simulink model "commhdlQPSKTxRxLoopback"  (R2025b)
settings: Solver=FixedStepDiscrete  StartTime=0.0  StopTime=stopTime  RelTol=1e-3
PostLoadFcn:
  | hScopeConfig = get_param([gcs '/Receiver/QPSK Rx/Frequency and Time Synchronizer/Symbol Synchronizer/No HDL/QPSK Receiver Eye Diagram'],'ScopeConfiguration');
  | 
  | hScopeConfig.OpenAtSimulationStart = false;
  | hScopeConfig.Visible = false;
  | SamplesPerSymbol = 4;
  | %UpsamplesRx = 1;
  | clear hScopeConfig
InitFcn:
  | commhdlQPSKTxRxModelInit;
  | % Rate bridge: ADRV9002/Jupiter radio runs at 15.36 MHz = 2x the 7.68 MHz
  | % (4 samples/symbol @ Rsym=1.92 MHz) the QPSK Rx requires. The deployed
  | % Receiver must downsample the ADC stream by 2. UpsamplesRx=1 fed the QPSK
  | % Rx 8 sps (2x-upsampled) and broke symbol sync / the loopback bit check.
  | UpsamplesRx = 2;
  | UpsamplesTx = 1;
  | clear simTimingOffset;
StopFcn:
  | if exist('simTimingOffset','var')
  |   disp('Simulation completed');
  |   %QPSKTxRxVerification;
  | end
values from neighbouring files (symbols this model uses):
  Rsym = variant{2}    [BandwidthVariantSimTest.m]    (also in CoarseFreqEstimatorTest.m = CoarseFreqEstimatorTest.Rsym; PreambleDetectorTest.m = 1920000)
undefined symbols (not defined in the file or in its folder): Add, Config, fsym, randsrc, RandStream, Shift
libraries: hdlsllib x149, simulink x40, dspsigops x36, dsphdlfiltering2 x6, dsphdlsigops2 x4, dsphdlmathfun2 x4, commdigbbndpm3 x4, commchan3 x1, commrflib2 x1
(part 6 of 6)

== system commhdlQPSKTxRxLoopback/TxRxLoopback/Receiver/QPSK Rx/Frequency and Time Synchronizer/Coarse Frequency Compensator/Coarse Frequency Estimator/Integrator ==
  note: store the value in the Reg before reset
  dataIn : Inport
  validIn : Inport  Port=2
  Add1 : Sum  Inputs=|++  OutDataTypeStr=Inherit: Same as first input
  Delay : Delay  DelayLength=1
  Delay1 : Delay  DelayLength=1
  Delay2 : Delay  DelayLength=1
  Integ Reg : hdlsllib/Discrete/Unit Delay Enabled Resettable Synchronous  InitialCondition=0.0  SampleTime=-1
  Reset Generator : Subsystem
  Store Reg : hdlsllib/Discrete/Unit Delay Enabled Synchronous  InitialCondition=0.0  SampleTime=-1
  IntegOut : Outport
  IntegValid : Outport  Port=2
  wires:
  Delay2/1 -> Integ Reg/2
  Reset Generator/1(reset) -> Integ Reg/3, Store Reg/2, Delay/1
  Store Reg/1 -> IntegOut/1
  Delay/1 -> IntegValid/1
  Delay1/1 -> Add1/1
  dataIn/1 -> Delay1/1
  validIn/1 -> Reset Generator/1(validIn), Delay2/1
  Integ Reg/1 -> Add1/2, Store Reg/1
  Add1/1 -> Integ Reg/1

== system commhdlQPSKTxRxLoopback/TxRxLoopback/Receiver/QPSK Rx/Frequency and Time Synchronizer/Phase Ambiguity Estimation and Correction/Phase Ambiguity Corrector/Reciprocal ==
  dataIn : Inport
  Compare To Constant : simulink/Logic and Bit Operations/Compare To Constant  relop=<  const=0  OutDataTypeStr=boolean
  Data Type Conversion : DataTypeConversion  OutDataTypeStr=fixdt(1,WL,0)  ConvertRealWorld=Stored Integer (SI)  SaturateOnIntegerOverflow=off  RndMeth=Floor
  Data Type Conversion1 : DataTypeConversion  OutDataTypeStr=fixdt(0,LUTAddrWL,0)  ConvertRealWorld=Stored Integer (SI)  SaturateOnIntegerOverflow=off  RndMeth=Floor
  Data Type Conversion2 : DataTypeConversion  OutDataTypeStr=fixdt(0,WL-LUTAddrWL,0)  ConvertRealWorld=Stored Integer (SI)  SaturateOnIntegerOverflow=off  RndMeth=Floor
  Delay : Delay  DelayLength=1
  Delay1 : Delay  DelayLength=1
  Delay2 : Delay  DelayLength=1
  Extract Bits : simulink/Logic and Bit Operations/Extract Bits  bitsToExtract=Range ending with least significant bit  numBits=LUTAddrWL  bitIdxRange=[0 7]  outScalingMode=Treat bit field as an integer
  Function Impl : Subsystem
  dataOut : Outport
  wires:
  Data Type Conversion2/1 -> Function Impl/1(switch)
  Delay2/1 -> Data Type Conversion1/1
  Delay1/1 -> Data Type Conversion2/1
  Delay/1 -> Extract Bits/1, Compare To Constant/1
  Function Impl/1(functionValues) -> dataOut/1
  Data Type Conversion1/1 -> Function Impl/2(LUTAddr)
  Compare To Constant/1 -> Delay1/1
  Data Type Conversion/1 -> Delay/1
  Extract Bits/1 -> Delay2/1
  dataIn/1 -> Data Type Conversion/1

== system commhdlQPSKTxRxLoopback/TxRxLoopback/Receiver/QPSK Rx/Frequency and Time Synchronizer/Phase Ambiguity Estimation and Correction/Phase Ambiguity Estimator/Subsystem ==
  L : Inport
  H : Inport  Port=2
  Delay6 : Delay  DelayLength=1  InitialCondition=1
  Logical Operator : Logic  AllPortsSameDT=off  OutDataTypeStr=boolean
  Logical Operator1 : Logic  Operator=NOT  IconShape=distinctive  AllPortsSameDT=off  OutDataTypeStr=boolean
  Logical Operator2 : Logic  Operator=OR  AllPortsSameDT=off  OutDataTypeStr=boolean
  Out2 : Outport
  wires:
  Logical Operator2/1 -> Delay6/1
  Logical Operator/1 -> Logical Operator2/2
  Logical Operator1/1 -> Logical Operator/1
  Delay6/1 -> Logical Operator/2, Out2/1
  H/1 -> Logical Operator2/1
  L/1 -> Logical Operator1/1

== system commhdlQPSKTxRxLoopback/TxRxLoopback/Receiver/QPSK Rx/Frequency and Time Synchronizer/Phase Ambiguity Estimation and Correction/Phase Ambiguity Estimator/Subsystem1 ==
  In1 : Inport
  validIn : Inport  Port=2
  Logical Operator1 : Logic  IconShape=distinctive  AllPortsSameDT=off  OutDataTypeStr=boolean
  Logical Operator2 : Logic  Operator=NOT  IconShape=distinctive  AllPortsSameDT=off  OutDataTypeStr=boolean
  validOut : Outport
  wires:
  Logical Operator2/1 -> Logical Operator1/1
  Logical Operator1/1 -> validOut/1
  validIn/1 -> Logical Operator1/2
  In1/1 -> Logical Operator2/1

== system commhdlQPSKTxRxLoopback/TxRxLoopback/Receiver/QPSK Rx/Frequency and Time Synchronizer/Preamble Detector/Correlator/Magnitude Squared ==
  In1 : Inport
  Delay1 : Delay
  Delay2 : Delay
  Delay3 : Delay
  Math Function : Math  Operator=conj
  Product : Product
  Out1 : Outport
  wires:
  Delay3/1 -> Out1/1
  Delay1/1 -> Product/2
  Delay2/1 -> Product/1
  Product/1 -> Delay3/1
  Math Function/1 -> Delay1/1
  In1/1 -> Delay2/1, Math Function/1

== system commhdlQPSKTxRxLoopback/TxRxLoopback/Receiver/QPSK Rx/Frequency and Time Synchronizer/Preamble Detector/Correlator/Magnitude Squared and Moving Sum ==
  scaled1 : Inport
  validIn : Inport  Port=2
  Add : Sum  Inputs=|+-  OutDataTypeStr=Inherit: Same as first input
  Add1 : Sum  Inputs=|++  OutDataTypeStr=Inherit: Same as first input
  Complex to Real-Imag1 : ComplexToRealImag  Output=Real
  Delay : Delay  DelayLength=13  ShowEnablePort=on
      settings: InputPortMap=u0,e6
  Delay{1..4,6,8..10,12} (9 alike) : Delay
  Delay11 : Delay  DelayLength=11
  Delay14 : Delay  DelayLength=1  ShowEnablePort=on
      settings: InputPortMap=u0,e6
  Delay5 : Delay  DelayLength=1
  Delay7 : Delay  DelayLength=1
  Gain : Gain  Gain=ThresoldGainFac  OutDataTypeStr=Inherit: Same as input
  Math Function1 : Math  Operator=conj
  Product1 : Product
  E1 : Outport
  wires:
  Delay12/1 -> Delay10/1
  Delay10/1 -> Delay9/1
  Delay9/1 -> Delay8/1
  Delay8/1 -> Delay7/1, Delay/2
  Delay7/1 -> Delay14/2
  Delay5/1 -> Add1/1
  Delay4/1 -> Add/1, Delay/1
  Delay3/1 -> Gain/1
  Delay2/1 -> Complex to Real-Imag1/1
  Delay1/1 -> Product1/2
  Delay6/1 -> Product1/1
  Gain/1 -> Delay4/1
  Product1/1 -> Delay2/1
  Math Function1/1 -> Delay1/1
  scaled1/1 -> Math Function1/1, Delay6/1
  Delay11/1 -> E1/1
  Add1/1 -> Delay14/1, Delay11/1
  Complex to Real-Imag1/1 -> Delay3/1
  Delay14/1 -> Add1/2
  Delay/1 -> Add/2
  validIn/1 -> Delay12/1
  Add/1 -> Delay5/1

== system commhdlQPSKTxRxLoopback/TxRxLoopback/Receiver/QPSK Rx/Frequency and Time Synchronizer/Preamble Detector/FIFO/Validate Input Push Pop ==
  rst : Inport
  push : Inport  Port=2
  pop : Inport  Port=3
  Compare To Constant : hdlsllib/Logic and Bit Operations/Compare To Constant  relop===  const=0  OutDataTypeStr=boolean
  Compare To Constant1 : hdlsllib/Logic and Bit Operations/Compare To Constant  relop===  const=fifoSize  OutDataTypeStr=boolean
  Constant : Constant  Value=true  SampleTime=-1
  Constant1 : Constant  Value=false  SampleTime=-1
  Delay : Delay  DelayLength=1
  Logical Operator1 : Logic  Operator=XOR  AllPortsSameDT=off  OutDataTypeStr=boolean
  Logical Operator2 : Logic  Operator=NOT  AllPortsSameDT=off  OutDataTypeStr=boolean
  Logical Operator{3..5,7,9} (5 alike) : Logic  AllPortsSameDT=off  OutDataTypeStr=boolean
  Logical Operator6 : Logic  Operator=NOT  AllPortsSameDT=off  OutDataTypeStr=boolean
  Logical Operator8 : Logic  Operator=NOT  AllPortsSameDT=off  OutDataTypeStr=boolean
  MATLAB Function : MATLAB Function  TreatAsAtomicUnit=on  mask{initVal=0, countToVal=fifoSize}
      mask prompts: initVal "Initial value:"; countToVal "Count to value:"
  No HDL : Subsystem
  Switch : Switch  Criteria=u2 ~= 0  SaturateOnIntegerOverflow=off  InputSameDT=off
  valid push : Outport
  valid pop : Outport  Port=2
  numEntries : Outport  Port=3
  wires:
  Delay/1 -> Compare To Constant/1, numEntries/1, Compare To Constant1/1
  rst/1 -> MATLAB Function/1(rst)
  Compare To Constant/1 -> Logical Operator3/1
  pop/1 -> Logical Operator7/1, Logical Operator3/2
  Switch/1 -> MATLAB Function/3(dir)
  MATLAB Function/1(count) -> Delay/1
  Constant1/1 -> Switch/1
  Logical Operator3/1 -> Logical Operator6/1, No HDL/2(popEmptyFIFO)  "pop on empty FIFO"
  Logical Operator4/1 -> Logical Operator2/1, No HDL/1(pushFullFIFO)  "push on full FIFO"
  Constant/1 -> Switch/3
  Compare To Constant1/1 -> Logical Operator4/2
  Logical Operator7/1 -> Logical Operator1/2, Logical Operator8/1, valid pop/1, Switch/2
  Logical Operator6/1 -> Logical Operator7/2
  Logical Operator1/1 -> MATLAB Function/2(enb)
  push/1 -> Logical Operator9/1, Logical Operator5/1
  Logical Operator8/1 -> Logical Operator5/2
  Logical Operator5/1 -> Logical Operator4/1
  Logical Operator2/1 -> Logical Operator9/2
  Logical Operator9/1 -> valid push/1, Logical Operator1/1

== system commhdlQPSKTxRxLoopback/TxRxLoopback/Receiver/QPSK Rx/Frequency and Time Synchronizer/Preamble Detector/Timing Adjust/No HDL ==
  note: This subsystem generates variables required for QPSKRxVerification for validation
  validIn : Inport
  timingOffset : Inport  Port=2
  syncPulse : Inport  Port=3
  Compare To Constant : simulink/Logic and Bit Operations/Compare To Constant  relop===  const=0  OutDataTypeStr=boolean
  Delay : Delay  DelayLength=4
  Delay1 : Delay  DelayLength=4
  Frame Counter : hdlsllib/Sources/HDL Counter  CountType=Free running  CountInit=0  CountStep=1  CountMax=bitsPerPacket/2 - 1  CountFromType=Initial value  CountFrom=0  CountResetPort=off  CountLoadPort=off  CountEnbPort=on  CountDirPort=off  CountHitOutputPort=off  CountDataType=Unsigned  CountWordLen=32  CountFracLen=0  CountSampTime=1
  Logical Operator : Logic  AllPortsSameDT=off  OutDataTypeStr=boolean
  No HDL : Subsystem
  No HDL1 : Subsystem
  Symbol Counter : hdlsllib/Sources/HDL Counter  CountType=Count limited  CountInit=0  CountStep=1  CountMax=bitsPerPacket/2 - 1  CountFromType=Initial value  CountFrom=0  CountResetPort=off  CountLoadPort=off  CountEnbPort=on  CountDirPort=off  CountHitOutputPort=off  CountDataType=Unsigned  CountWordLen=nextpow2(bitsPerPacket/2 - 1)  CountFracLen=0  CountSampTime=1
  Unit Delay Enabled Synchronous : hdlsllib/Discrete/Unit Delay Enabled Synchronous  InitialCondition=0.0  SampleTime=-1
  wires:
  Delay1/1 -> No HDL/1(timingOffset)
  Delay/1 -> No HDL1/Enable, No HDL/Enable
  Unit Delay Enabled Synchronous/1 -> No HDL1/1(frameNumber)
  syncPulse/1 -> Delay/1
  Frame Counter/1 -> Unit Delay Enabled Synchronous/1
  Compare To Constant/1 -> Logical Operator/1
  Logical Operator/1 -> Frame Counter/1, Unit Delay Enabled Synchronous/2
  Symbol Counter/1 -> Compare To Constant/1
  validIn/1 -> Symbol Counter/1, Logical Operator/2
  timingOffset/1 -> Delay1/1

== system commhdlQPSKTxRxLoopback/TxRxLoopback/Receiver/QPSK Rx/Frequency and Time Synchronizer/Symbol Synchronizer/Gardner TED/GTED ==
  In1 : Inport
  Add : Sum
  Add1 : Sum  Inputs=+-
  Add2 : Sum  Inputs=+-
  Complex to Real-Imag : ComplexToRealImag
  Delay{,1..7} (8 alike) : Delay  DelayLength=1
  Delay{8..13} (6 alike) : Delay
  Product : Product
  Product1 : Product
  Out1 : Outport
  wires:
  Delay13/1 -> Add/2
  Delay12/1 -> Product1/2
  Delay11/1 -> Product1/1
  Delay10/1 -> Add/1
  Delay9/1 -> Product/2
  Delay8/1 -> Product/1
  Complex to Real-Imag/2 -> Delay4/1, Add2/2
  Delay7/1 -> Add2/1
  Delay4/1 -> Delay5/1
  Delay6/1 -> Delay7/1
  Add2/1 -> Delay12/1
  Delay5/1 -> Delay6/1, Delay11/1
  Delay1/1 -> Delay8/1, Delay2/1
  Add1/1 -> Delay9/1
  Delay2/1 -> Delay3/1
  Delay/1 -> Delay1/1
  Delay3/1 -> Add1/1
  Complex to Real-Imag/1 -> Delay/1, Add1/2
  In1/1 -> Complex to Real-Imag/1
  Add/1 -> Out1/1
  Product1/1 -> Delay13/1
  Product/1 -> Delay10/1

== system commhdlQPSKTxRxLoopback/TxRxLoopback/Receiver/QPSK Rx/Frequency and Time Synchronizer/Symbol Synchronizer/No HDL/No HDL ==
  data : Inport
  Enable : EnablePort
  Data Type Conversion : DataTypeConversion  OutDataTypeStr=double  SaturateOnIntegerOverflow=off  RndMeth=Floor
  wires:
  data/1 -> Data Type Conversion/1
  Data Type Conversion/1 -> ?

== system commhdlQPSKTxRxLoopback/TxRxLoopback/Receiver/QPSK Rx/Frequency and Time Synchronizer/Symbol Synchronizer/Rate Handle/FIFO ==
  in : Inport
  push : Inport  Port=2
  pop : Inport  Port=3
  reset : Inport  Port=4
  Delay1 : Delay  DelayLength=1
  Pop Counter : hdlsllib/Sources/HDL Counter  CountType=Count limited  CountInit=0  CountStep=1  CountMax=fifoSize -1  CountFromType=Initial value  CountFrom=0  CountResetPort=on  CountLoadPort=off  CountEnbPort=on  CountDirPort=off  CountHitOutputPort=off  CountDataType=Unsigned  CountWordLen=nextpow2(fifoSize)  CountFracLen=0  CountSampTime=1
  Push Counter : hdlsllib/Sources/HDL Counter  CountType=Count limited  CountInit=0  CountStep=1  CountMax=fifoSize -1  CountFromType=Initial value  CountFrom=0  CountResetPort=on  CountLoadPort=off  CountEnbPort=on  CountDirPort=off  CountHitOutputPort=off  CountDataType=Unsigned  CountWordLen=nextpow2(fifoSize)  CountFracLen=0  CountSampTime=1
  Simple Dual Port RAM : hdlsllib/HDL RAMs/Simple Dual Port RAM  ram_size=nextpow2(fifoSize)
  Validate Input Push Pop : Subsystem
  out : Outport
  numEntries : Outport  Port=2
  validPop : Outport  Port=3
  wires:
  Validate Input Push Pop/3(numEntries) -> numEntries/1
  Simple Dual Port RAM/1 -> out/1
  Push Counter/1 -> Simple Dual Port RAM/2
  Pop Counter/1 -> Simple Dual Port RAM/4
  push/1 -> Validate Input Push Pop/2(push)
  pop/1 -> Validate Input Push Pop/3(pop)
  Validate Input Push Pop/1(valid push) -> Simple Dual Port RAM/3, Push Counter/2
  Validate Input Push Pop/2(valid pop) -> validPop/1, Pop Counter/2
  reset/1 -> Delay1/1, Validate Input Push Pop/1(rst)
  in/1 -> Simple Dual Port RAM/1
  Delay1/1 -> Pop Counter/1, Push Counter/1

== system commhdlQPSKTxRxLoopback/TxRxLoopback/Transmitter/QPSK Tx/Bit Packetizer/Data Bits FIFO/No HDL/No HDL ==
  push : Inport
  full : Inport  Port=2
  ncount : Inport  Port=3
  empty : Inport  Port=4
  pop : Inport  Port=5
  Assertion : Assertion
  Assertion1 : Assertion
  Display : Display
  Logical Operator : Logic  Operator=NAND  AllPortsSameDT=off  OutDataTypeStr=boolean
  Logical Operator1 : Logic  Operator=NAND  AllPortsSameDT=off  OutDataTypeStr=boolean
  wires:
  push/1 -> Logical Operator/1
  empty/1 -> Logical Operator1/1
  full/1 -> Logical Operator/2
  pop/1 -> Logical Operator1/2
  Logical Operator/1 -> Assertion/1
  ncount/1 -> Display/1
  Logical Operator1/1 -> Assertion1/1

== system commhdlQPSKTxRxLoopback/Receiver/QPSK Rx/Frequency and Time Synchronizer/Symbol Synchronizer/Rate Handle/FIFO/Validate Input Push Pop/No HDL ==
  pushFullFIFO : Inport
  popEmptyFIFO : Inport  Port=2
  Constant2 : Constant  Value=pushFullDiag  SampleTime=-1
  Constant3 : Constant  Value=popEmptyDiag  SampleTime=-1
  MATLAB Function : MATLAB Function  TreatAsAtomicUnit=on
  wires:
  Constant2/1 -> MATLAB Function/1(pushFullDiag)
  Constant3/1 -> MATLAB Function/2(popEmptyDiag)
  popEmptyFIFO/1 -> MATLAB Function/4(popEmpty)
  pushFullFIFO/1 -> MATLAB Function/3(pushFull)

== system commhdlQPSKTxRxLoopback/TxRxLoopback/Receiver/QPSK Rx/Frequency and Time Synchronizer/Coarse Frequency Compensator/Coarse Frequency Estimator/Integrator/Reset Generator ==
  validIn : Inport
  Compare To Constant : simulink/Logic and Bit Operations/Compare To Constant  relop===  const=integAvgLen  OutDataTypeStr=boolean
  Delay1 : Delay  DelayLength=1
  Delay5 : Delay  DelayLength=1
  HDL Counter : hdlsllib/Sources/HDL Counter  CountType=Count limited  CountInit=0  CountStep=1  CountMax=integAvgLen  CountFromType=Initial value  CountFrom=0  CountResetPort=off  CountLoadPort=off  CountEnbPort=on  CountDirPort=off  CountHitOutputPort=off  CountDataType=Unsigned  CountWordLen=nextpow2(integAvgLen + 1)  CountFracLen=0  CountSampTime=1
  Logical Operator : Logic  AllPortsSameDT=off  OutDataTypeStr=boolean
  reset : Outport
  wires:
  HDL Counter/1 -> Delay5/1
  Compare To Constant/1 -> Logical Operator/2
  validIn/1 -> Delay1/1, HDL Counter/1
  Logical Operator/1 -> reset/1
  Delay5/1 -> Compare To Constant/1
  Delay1/1 -> Logical Operator/1

== system commhdlQPSKTxRxLoopback/TxRxLoopback/Receiver/QPSK Rx/Frequency and Time Synchronizer/Phase Ambiguity Estimation and Correction/Phase Ambiguity Corrector/Reciprocal/Function Impl ==
  switch : Inport
  LUTAddr : Inport  Port=2
  Delay{6..8,10,15..16} (6 alike) : Delay
  Delay9 : Delay  DelayLength=1
  LUT1 : LookupNDDirect  NumberOfTableDimensions=1  Table=LUT(:,1)  DiagnosticForOutOfRangeInput=Error
  LUT2 : LookupNDDirect  NumberOfTableDimensions=1  Table=LUT(:,2)  DiagnosticForOutOfRangeInput=Error
  Multiport Switch : MultiPortSwitch  DataPortOrder=Zero-based contiguous  Inputs=2  zeroidx=on  SaturateOnIntegerOverflow=off  InputSameDT=off
  functionValues : Outport
  wires:
  LUTAddr/1 -> Delay7/1, Delay6/1
  Delay15/1 -> Multiport Switch/2
  Delay16/1 -> Multiport Switch/3
  Delay10/1 -> Multiport Switch/1
  Delay9/1 -> functionValues/1
  LUT2/1 -> Delay15/1
  LUT1/1 -> Delay16/1
  switch/1 -> Delay8/1
  Delay8/1 -> Delay10/1
  Delay7/1 -> LUT2/1
  Delay6/1 -> LUT1/1
  Multiport Switch/1 -> Delay9/1

== system commhdlQPSKTxRxLoopback/TxRxLoopback/Receiver/QPSK Rx/Frequency and Time Synchronizer/Preamble Detector/FIFO/Validate Input Push Pop/No HDL ==
  pushFullFIFO : Inport
  popEmptyFIFO : Inport  Port=2
  Constant2 : Constant  Value=pushFullDiag  SampleTime=-1
  Constant3 : Constant  Value=popEmptyDiag  SampleTime=-1
  MATLAB Function : MATLAB Function  TreatAsAtomicUnit=on
  wires:
  pushFullFIFO/1 -> MATLAB Function/3(pushFull)
  popEmptyFIFO/1 -> MATLAB Function/4(popEmpty)
  Constant3/1 -> MATLAB Function/2(popEmptyDiag)
  Constant2/1 -> MATLAB Function/1(pushFullDiag)

== system commhdlQPSKTxRxLoopback/TxRxLoopback/Receiver/QPSK Rx/Frequency and Time Synchronizer/Preamble Detector/Timing Adjust/No HDL/No HDL ==
  timingOffset : Inport
  Enable : EnablePort
  Data Type Conversion : DataTypeConversion  OutDataTypeStr=double  SaturateOnIntegerOverflow=off  RndMeth=Floor
  wires:
  timingOffset/1 -> Data Type Conversion/1
  Data Type Conversion/1 -> ?

== system commhdlQPSKTxRxLoopback/TxRxLoopback/Receiver/QPSK Rx/Frequency and Time Synchronizer/Preamble Detector/Timing Adjust/No HDL/No HDL1 ==
  frameNumber : Inport
  Enable : EnablePort
  Data Type Conversion : DataTypeConversion  OutDataTypeStr=double  SaturateOnIntegerOverflow=off  RndMeth=Floor
  wires:
  Data Type Conversion/1 -> ?
  frameNumber/1 -> Data Type Conversion/1

== system commhdlQPSKTxRxLoopback/TxRxLoopback/Receiver/QPSK Rx/Frequency and Time Synchronizer/Symbol Synchronizer/Rate Handle/FIFO/Validate Input Push Pop ==
  rst : Inport
  push : Inport  Port=2
  pop : Inport  Port=3
  Compare To Constant : hdlsllib/Logic and Bit Operations/Compare To Constant  relop===  const=0  OutDataTypeStr=boolean
  Compare To Constant1 : hdlsllib/Logic and Bit Operations/Compare To Constant  relop===  const=fifoSize  OutDataTypeStr=boolean
  Constant : Constant  Value=true  SampleTime=-1
  Constant1 : Constant  Value=false  SampleTime=-1
  Delay : Delay  DelayLength=1
  Logical Operator1 : Logic  Operator=XOR  AllPortsSameDT=off  OutDataTypeStr=boolean
  Logical Operator2 : Logic  Operator=NOT  AllPortsSameDT=off  OutDataTypeStr=boolean
  Logical Operator{3..5,7,9} (5 alike) : Logic  AllPortsSameDT=off  OutDataTypeStr=boolean
  Logical Operator6 : Logic  Operator=NOT  AllPortsSameDT=off  OutDataTypeStr=boolean
  Logical Operator8 : Logic  Operator=NOT  AllPortsSameDT=off  OutDataTypeStr=boolean
  MATLAB Function : MATLAB Function  TreatAsAtomicUnit=on  mask{initVal=0, countToVal=fifoSize}
      mask prompts: initVal "Initial value:"; countToVal "Count to value:"
  No HDL : Subsystem
  Switch : Switch  Criteria=u2 ~= 0  SaturateOnIntegerOverflow=off  InputSameDT=off
  valid push : Outport
  valid pop : Outport  Port=2
  numEntries : Outport  Port=3
  wires:
  Delay/1 -> Compare To Constant/1, numEntries/1, Compare To Constant1/1
  rst/1 -> MATLAB Function/1(rst)
  Compare To Constant/1 -> Logical Operator3/1
  pop/1 -> Logical Operator7/1, Logical Operator3/2
  Switch/1 -> MATLAB Function/3(dir)
  MATLAB Function/1(count) -> Delay/1
  Constant1/1 -> Switch/1
  Logical Operator3/1 -> Logical Operator6/1, No HDL/2(popEmptyFIFO)  "pop on empty FIFO"
  Logical Operator4/1 -> Logical Operator2/1, No HDL/1(pushFullFIFO)  "push on full FIFO"
  Constant/1 -> Switch/3
  Compare To Constant1/1 -> Logical Operator4/2
  Logical Operator7/1 -> Logical Operator1/2, Logical Operator8/1, valid pop/1, Switch/2
  Logical Operator6/1 -> Logical Operator7/2
  Logical Operator1/1 -> MATLAB Function/2(enb)
  push/1 -> Logical Operator9/1, Logical Operator5/1
  Logical Operator8/1 -> Logical Operator5/2
  Logical Operator5/1 -> Logical Operator4/1
  Logical Operator2/1 -> Logical Operator9/2
  Logical Operator9/1 -> valid push/1, Logical Operator1/1

== system commhdlQPSKTxRxLoopback/TxRxLoopback/Receiver/QPSK Rx/Frequency and Time Synchronizer/Symbol Synchronizer/Rate Handle/FIFO/Validate Input Push Pop/No HDL ==
  pushFullFIFO : Inport
  popEmptyFIFO : Inport  Port=2
  Constant2 : Constant  Value=pushFullDiag  SampleTime=-1
  Constant3 : Constant  Value=popEmptyDiag  SampleTime=-1
  MATLAB Function : MATLAB Function  TreatAsAtomicUnit=on
  wires:
  pushFullFIFO/1 -> MATLAB Function/3(pushFull)
  popEmptyFIFO/1 -> MATLAB Function/4(popEmpty)
  Constant3/1 -> MATLAB Function/2(popEmptyDiag)
  Constant2/1 -> MATLAB Function/1(pushFullDiag)

== matlab function commhdlQPSKTxRxLoopback/Receiver/Capture Data Bits/MATLAB Function ==
  data: valid input; datain input; start input; stop input; count_out output; packets_out output; bit_errors_out output
function [count_out, packets_out, bit_errors_out] = msgdec(valid, datain, start, stop)

persistent count;
persistent msgbuffer;

persistent packetsReceived
persistent errors;

if isempty(count) || isempty(msgbuffer) || isempty(packetsReceived)
    count = uint32(0);
    msgbuffer = zeros(1,120+8)>0; % ADI Hello WorldX
    packetsReceived = uint32(0);
    errors = uint32(0);
end

% Mesg
strAscii = dec2bin('ADI Hello World',8);
msgarray = reshape(strAscii', [1, numel(strAscii)]);
msgbits = logical(msgarray - 48);

% msgLen = uint32(2240);

if valid
    if start
        count = uint32(1);
        packetsReceived = packetsReceived + 1;
    end

    if count <= (length(msgbuffer) - 8)
        msgbuffer(count) = datain;
        if datain ~= msgbits(count)
            errors = errors + 1;
        end

    elseif count == length(msgbuffer) + 1
        msgarray_dec = char('0' + msgbuffer);
        N = length(msgarray_dec) / 8;
        strAscii_dec = reshape(msgarray_dec , 8, N).';
        msg = char(bin2dec(strAscii_dec).');
        disp(msg);
    end
    
    if count <= length(msgbuffer) + 2
        count = count + 1;
    end
end

count_out = count;
packets_out = packetsReceived;
bit_errors_out = errors;

== matlab function commhdlQPSKTxRxLoopback/TxRxLoopback/Transmitter/Input Data/Message Generator/MATLAB Function ==
  data: enable input; reset input; out output; start output; stop output; valid output; count_out output; msg_count_out output
function [out, start, stop, valid, count_out, msg_count_out] = msggen(enable, reset)

persistent indexCount;
persistent toggle;
persistent msgCount;
persistent msgCountAll;
persistent msgCountBitIndex;

if isempty(indexCount) || isempty(toggle) || isempty(msgCount) || isempty(msgCountBitIndex) || isempty(msgCountAll)
    indexCount = uint32(0);
    msgCount = uint32(1);
    msgCountAll = uint32(1);
    msgCountBitIndex = uint8(0);
    toggle = false;
end

%% Constants
strAscii = dec2bin('ADI Hello World', 8);
msgarray = reshape(strAscii', [1, numel(strAscii)]);
msgbits = logical(msgarray - 48);
msgbitsLen = length(msgbits);

fullMessageLen = uint32(2240-1); % Need the -1 to eat the feedback delay

% Bit counter
% N = 8;% 8-bit counter
% mask = uint32(2^N - 1);
% for k = 1:300
%     msgCount = bitand(msgCount + uint32(1), mask);   % wraps 255 -> 0
% end

%% Logic
if enable && ~reset
    % Set out data
    if indexCount < msgbitsLen % Insert msg
        out = msgbits(indexCount + 1);
        msgCountBitIndex = uint8(0);
    elseif msgCountBitIndex < (8) % Number insert
        out = bitget(msgCount+48, 8-msgCountBitIndex) > 0;
        msgCountBitIndex = msgCountBitIndex + 1;
    else % Toggle bits after message
        out = toggle;
        msgCountBitIndex = uint8(0);
        if toggle
            toggle = false;
        else
            toggle = true;
        end
    end

    % Flags
    start = indexCount == uint32(0);
    stop = indexCount == fullMessageLen;
    valid = true;

    % Counters
    if fullMessageLen == indexCount
        if msgCount >= 9
            msgCount = uint32(1);
        else
            msgCount = msgCount +  1;
            msgCountAll = msgCountAll + 1;
        end
    end
    if indexCount <= fullMessageLen
        indexCount = indexCount + 1;
    end

else % Enable == false

    if reset
        indexCount = uint32(0);
        % msgCount = uint32(0);
        msgCountBitIndex = uint8(0);
        toggle = false;
    end
    out = false;
    start = false;
    stop = false;
    valid = false;
end

if isempty(indexCount)
    count_out = uint32(0);
else
    count_out = indexCount;
end

msg_count_out = msgCountAll;

== matlab function commhdlQPSKTxRxLoopback/Receiver/QPSK Rx/Frequency and Time Synchronizer/Preamble Detector/FIFO/Validate Input Push Pop/MATLAB Function ==
  data: rst input; count output; enb input; dir input; initVal parameter; countToVal parameter
function count = hdlCounter(rst,enb,dir,initVal,countToVal)
%#codegen

persistent countReg

if(isempty(countReg))
    countReg = fi(initVal,0,nextpow2(countToVal+1),0);
end

if(rst)
    countReg(:) = initVal;
elseif(enb)
    if(dir)
        if(countReg==countToVal)
            countReg(:) = initVal;
        else
            countReg(:) = countReg+1;
        end
    else
        if(countReg==initVal)
            countReg(:) = countToVal;
        else
            countReg(:) = countReg-1;
        end
    end
end

count = countReg;

end

== matlab function commhdlQPSKTxRxLoopback/Receiver/QPSK Rx/Frequency and Time Synchronizer/Preamble Detector/FIFO/Validate Input Push Pop/No HDL/MATLAB Function ==
  data: pushFullDiag input; popEmptyDiag input; pushFull input; popEmpty input
function pushPopDiagnostics(pushFullDiag, popEmptyDiag, pushFull, popEmpty)
%#codegen


if(pushFull)
    switch pushFullDiag
        case 2
            warning('Push signal applied on full FIFO');
        case 3
            error('Push signal applied on full FIFO');
        otherwise
    end
end

if(popEmpty)
    switch popEmptyDiag
        case 2
            warning('Pop signal applied on empty FIFO');
        case 3
            error('Pop signal applied on empty FIFO');
        otherwise
    end
end

end

== matlab function commhdlQPSKTxRxLoopback/TxRxLoopback/Transmitter/QPSK Tx/Bit Packetizer/Data Bits FIFO/MATLAB Function1 ==
  data: wr input; full output; rd input; dataBitsPerPacket parameter
function full = fcn(wr,rd,dataBitsPerPacket)
%#codegen
     
    depth = dataBitsPerPacket*2 - 1;
    persistent count;
    if isempty(count)
        count = fi(0,0,nextpow2(depth),0,hdlfimath);
    end

    if wr
        count(:) = count + 1;
    end
    if rd
        count(:) = count - 1;
    end

    full = (count > depth);

end

== matlab function commhdlQPSKTxRxLoopback/Transmitter/QPSK Tx/Bit Packetizer/Data Bits FIFO/No HDL/MATLAB Function ==
  data: wr input; full output; rd input; ncount output; empty output; dataBitsPerPacket parameter
function [full,ncount,empty] = fcn(wr,rd,dataBitsPerPacket)
%#codegen
     
    depth = dataBitsPerPacket*2 - 1;
    persistent count;
    if isempty(count)
        count = fi(0,0,nextpow2(depth),0,hdlfimath);
    end

    empty = (count == 0);
    full = (count > depth);
    ncount = count;

    if wr
        count(:) = count + 1;
    end
    if rd
        count(:) = count - 1;
    end

end

== matlab function commhdlQPSKTxRxLoopback/TxRxLoopback/Transmitter/QPSK Tx/Bit Packetizer/Data Bits FIFO/No HDL/MATLAB Function ==
  data: wr input; full output; rd input; ncount output; empty output; dataBitsPerPacket parameter
function [full,ncount,empty] = fcn(wr,rd,dataBitsPerPacket)
%#codegen
     
    depth = dataBitsPerPacket*2 - 1;
    persistent count;
    if isempty(count)
        count = fi(0,0,nextpow2(depth),0,hdlfimath);
    end

    empty = (count == 0);
    full = (count > depth);
    ncount = count;

    if wr
        count(:) = count + 1;
    end
    if rd
        count(:) = count - 1;
    end

end

== matlab function commhdlQPSKTxRxLoopback/Receiver/QPSK Rx/Frequency and Time Synchronizer/Packet Controller/MATLAB Function ==
  data: valid input; syncPulse input; out output
function out = fcn(valid,syncPulse)
%#codegen

  persistent Reg;
  if isempty(Reg)
      Reg = false;
  end
  
  out = Reg;
  
  if Reg && valid
      Reg = false;
  end
  
  if syncPulse
      Reg = true;
  end
  
end

== matlab function commhdlQPSKTxRxLoopback/TxRxLoopback/Transmitter/QPSK Tx/Bit Packetizer/Data Bits FIFO/RAM Frame Status Indicator ==
  data: push input; out output; pop input; dataBitsPerPacket parameter
function out = fcn(push,pop,dataBitsPerPacket)

   persistent pushCount popCount frameCount;
   if isempty(pushCount)
       pushCount = fi(0,0,nextpow2(dataBitsPerPacket),0,hdlfimath);
       frameCount = fi(0,0,2,0,hdlfimath);
       popCount = fi(0,0,nextpow2(dataBitsPerPacket),0,hdlfimath);
   end
   
   if (pushCount == dataBitsPerPacket-1) && push
       frameCount(:) = frameCount + 1;
   end
   if (popCount == dataBitsPerPacket-1) && pop
       frameCount(:) = frameCount - 1;
   end

   if push
       if pushCount == dataBitsPerPacket - 1
           pushCount(:) = 0;
       else
           pushCount(:) = pushCount + 1;
       end
   end

   if pop 
       if popCount == dataBitsPerPacket - 1
           popCount(:) = 0;
       else
           popCount(:) = popCount + 1;
       end
   end

   out = frameCount;

end

== matlab function commhdlQPSKTxRxLoopback/TxRxLoopback/Receiver/Capture Data Bits/MATLAB Function ==
  data: valid input; datain input; start input; stop input; count_out output; packets_out output; bit_errors_out output
function [count_out, packets_out, bit_errors_out] = msgdec(valid, datain, start, stop)

persistent count;
persistent msgbuffer;

persistent packetsReceived
persistent errors;

if isempty(count) || isempty(msgbuffer) || isempty(packetsReceived)
    count = uint32(0);
    msgbuffer = zeros(1,120+8)>0; % ADI Hello WorldX
    packetsReceived = uint32(0);
    errors = uint32(0);
end

% Mesg
strAscii = dec2bin('ADI Hello World',8);
msgarray = reshape(strAscii', [1, numel(strAscii)]);
msgbits = logical(msgarray - 48);

% msgLen = uint32(2240);

if valid
    if start
        count = uint32(1);
        packetsReceived = packetsReceived + 1;
    end

    if count <= (length(msgbuffer) - 8)
        msgbuffer(count) = datain;
        if datain ~= msgbits(count)
            errors = errors + 1;
        end

    elseif count == length(msgbuffer) + 1
        msgarray_dec = char('0' + msgbuffer);
        N = length(msgarray_dec) / 8;
        strAscii_dec = reshape(msgarray_dec , 8, N).';
        msg = char(bin2dec(strAscii_dec).');
        disp(msg);
    end
    
    if count <= length(msgbuffer) + 2
        count = count + 1;
    end
end

count_out = count;
packets_out = packetsReceived;
bit_errors_out = errors;

== matlab function commhdlQPSKTxRxLoopback/TxRxLoopback/Receiver/QPSK Rx/Frequency and Time Synchronizer/Packet Controller/MATLAB Function ==
  data: valid input; syncPulse input; out output
function out = fcn(valid,syncPulse)
%#codegen

  persistent Reg;
  if isempty(Reg)
      Reg = false;
  end
  
  out = Reg;
  
  if Reg && valid
      Reg = false;
  end
  
  if syncPulse
      Reg = true;
  end
  
end

== matlab function commhdlQPSKTxRxLoopback/TxRxLoopback/Receiver/QPSK Rx/Frequency and Time Synchronizer/Packet Controller/sample discard controller ==
  data: dataIn input; validIn input; dataOut output; startIn input; endIn input; startOut output; endOut output; validOut output
function [dataOut,startOut,endOut,validOut] = controller(dataIn,validIn,startIn,endIn)
%#codegen

   persistent active dataOutReg validOutReg startOutReg endOutReg;
   if isempty(active)
      active  = false;
      dataOutReg = cast(0,'like',dataIn);
      validOutReg = false;
      startOutReg = false;
      endOutReg = false;
   end
   
   dataOut = dataOutReg;
   validOut = validOutReg;
   startOut = startOutReg;
   endOut = endOutReg;
   
   startOutReg = startIn;
   endOutReg = endIn;
   
   if startIn
       active = true;
   end
   
   if active
       dataOutReg(:) = dataIn;
       validOutReg = validIn;
   else
       dataOutReg(:) = 0;
       validOutReg = false;
   end
   
   if endIn
       if active 
           endOutReg = true;
       else
           endOutReg = false;
       end
       active = false;
   end
end

== matlab function commhdlQPSKTxRxLoopback/TxRxLoopback/Receiver/QPSK Rx/Frequency and Time Synchronizer/Preamble Detector/Correlator/ThresholdLimiter ==
  settings: fimath=hdlfimath
  data: x input; y output
function y = applyLowerLimit(x)
    % Apply a lower limit to the threshold.
    %#codegen
    
    % Threshold is computed by summing across 63 samples.
    % Set lower limit to be equivalent of all 63 samples
    % having their LSB set to 1 and all others set to 0. 
    lowerLimit = cast(0.01, 'like', x);
    
    if x < lowerLimit
        y = lowerLimit;
    else
        y = x;
    end
end

== matlab function commhdlQPSKTxRxLoopback/TxRxLoopback/Receiver/QPSK Rx/Frequency and Time Synchronizer/Preamble Detector/FIFO/Validate Input Push Pop/MATLAB Function ==
  data: rst input; count output; enb input; dir input; initVal parameter; countToVal parameter
function count = hdlCounter(rst,enb,dir,initVal,countToVal)
%#codegen

persistent countReg

if(isempty(countReg))
    countReg = fi(initVal,0,nextpow2(countToVal+1),0);
end

if(rst)
    countReg(:) = initVal;
elseif(enb)
    if(dir)
        if(countReg==countToVal)
            countReg(:) = initVal;
        else
            countReg(:) = countReg+1;
        end
    else
        if(countReg==initVal)
            countReg(:) = countToVal;
        else
            countReg(:) = countReg-1;
        end
    end
end

count = countReg;

end

== matlab function commhdlQPSKTxRxLoopback/TxRxLoopback/Receiver/QPSK Rx/Frequency and Time Synchronizer/Preamble Detector/FIFO/Validate Input Push Pop/No HDL/MATLAB Function ==
  data: pushFullDiag input; popEmptyDiag input; pushFull input; popEmpty input
function pushPopDiagnostics(pushFullDiag, popEmptyDiag, pushFull, popEmpty)
%#codegen


if(pushFull)
    switch pushFullDiag
        case 2
            warning('Push signal applied on full FIFO');
        case 3
            error('Push signal applied on full FIFO');
        otherwise
    end
end

if(popEmpty)
    switch popEmptyDiag
        case 2
            warning('Pop signal applied on empty FIFO');
        case 3
            error('Pop signal applied on empty FIFO');
        otherwise
    end
end

end

== matlab function commhdlQPSKTxRxLoopback/TxRxLoopback/Receiver/QPSK Rx/Frequency and Time Synchronizer/Symbol Synchronizer/Interpolation Control ==
  data: mu output; Delta input; Underflow output
function [mu,Underflow] = Interpolation_ctrl(Delta)
% Implementation of modulo-1 counter for interpolation control listed in
% Figure 8.4.19 of "Digital Communications - A Discrete-Time Approach"
% by Michael Rice. See design details in Chapter 8.4.3 of the same book.
% 
% Input:
%   Delta - Loop filter output. If loop is in lock, delta would be small
% Output:
%   Underflow - Indicator of counter underflow. This is the strobe signal
%               for downstream processing
%   mu - Difference between actual sampling instant and the optimal instant,
%        between zero and one
%#codegen

% countReg - Counter value delayed by 1 sample
% muReg - The estimated timing error normalized by half QPSK symbols

   mask = fi(1-2^(-10),1,11,10);
   
   persistent countReg underflowReg muReg;
   if isempty(countReg)
       countReg  = fi(0,1,11,10);
       muReg = fi(0,1,11,10);
       underflowReg = false;
   end
   
   
   Underflow = underflowReg;
   mu = muReg;   
   
   
   counter = bitand(mask,countReg)-Delta-fi(0.25,1,11,10); % decrementing counter
   
   % if countReg is a nonnegative number,
   % then mod(countReg,1) equals the fractional part of countReg
   if counter < 0
       underflowReg = true;
       muReg = bitshift(bitand(mask,countReg),2);
       countReg = fi(counter+1,1,11,10);% create underflow to counter
   else
       underflowReg = false;
       countReg = fi(counter,1,11,10);
   end
   


end

== matlab function commhdlQPSKTxRxLoopback/Receiver/QPSK Rx/Frequency and Time Synchronizer/Symbol Synchronizer/Rate Handle/FIFO/Validate Input Push Pop/MATLAB Function ==
  data: rst input; count output; enb input; dir input; initVal parameter; countToVal parameter
function count = hdlCounter(rst,enb,dir,initVal,countToVal)
%#codegen

persistent countReg

if(isempty(countReg))
    countReg = fi(initVal,0,nextpow2(countToVal+1),0);
end

if(rst)
    countReg(:) = initVal;
elseif(enb)
    if(dir)
        if(countReg==countToVal)
            countReg(:) = initVal;
        else
            countReg(:) = countReg+1;
        end
    else
        if(countReg==initVal)
            countReg(:) = countToVal;
        else
            countReg(:) = countReg-1;
        end
    end
end

count = countReg;

end

== matlab function commhdlQPSKTxRxLoopback/TxRxLoopback/Receiver/QPSK Rx/Frequency and Time Synchronizer/Symbol Synchronizer/Rate Handle/FIFO/Validate Input Push Pop/MATLAB Function ==
  data: rst input; count output; enb input; dir input; initVal parameter; countToVal parameter
function count = hdlCounter(rst,enb,dir,initVal,countToVal)
%#codegen

persistent countReg

if(isempty(countReg))
    countReg = fi(initVal,0,nextpow2(countToVal+1),0);
end

if(rst)
    countReg(:) = initVal;
elseif(enb)
    if(dir)
        if(countReg==countToVal)
            countReg(:) = initVal;
        else
            countReg(:) = countReg+1;
        end
    else
        if(countReg==initVal)
            countReg(:) = countToVal;
        else
            countReg(:) = countReg-1;
        end
    end
end

count = countReg;

end

== matlab function commhdlQPSKTxRxLoopback/TxRxLoopback/Receiver/QPSK Rx/Frequency and Time Synchronizer/Symbol Synchronizer/Rate Handle/FIFO/Validate Input Push Pop/No HDL/MATLAB Function ==
  data: pushFullDiag input; popEmptyDiag input; pushFull input; popEmpty input
function pushPopDiagnostics(pushFullDiag, popEmptyDiag, pushFull, popEmpty)
%#codegen


if(pushFull)
    switch pushFullDiag
        case 2
            warning('Push signal applied on full FIFO');
        case 3
            error('Push signal applied on full FIFO');
        otherwise
    end
end

if(popEmpty)
    switch popEmptyDiag
        case 2
            warning('Pop signal applied on empty FIFO');
        case 3
            error('Pop signal applied on empty FIFO');
        otherwise
    end
end

end

== matlab function commhdlQPSKTxRxLoopback/Transmitter/QPSK Tx/Bit Packetizer/Data Bits FIFO/MATLAB Function1 ==
  data: wr input; full output; rd input; dataBitsPerPacket parameter
function full = fcn(wr,rd,dataBitsPerPacket)
%#codegen
     
    depth = dataBitsPerPacket*2 - 1;
    persistent count;
    if isempty(count)
        count = fi(0,0,nextpow2(depth),0,hdlfimath);
    end

    if wr
        count(:) = count + 1;
    end
    if rd
        count(:) = count - 1;
    end

    full = (count > depth);

end

== matlab function commhdlQPSKTxRxLoopback/Transmitter/QPSK Tx/Bit Packetizer/Data Bits FIFO/RAM Frame Status Indicator ==
  data: push input; out output; pop input; dataBitsPerPacket parameter
function out = fcn(push,pop,dataBitsPerPacket)

   persistent pushCount popCount frameCount;
   if isempty(pushCount)
       pushCount = fi(0,0,nextpow2(dataBitsPerPacket),0,hdlfimath);
       frameCount = fi(0,0,2,0,hdlfimath);
       popCount = fi(0,0,nextpow2(dataBitsPerPacket),0,hdlfimath);
   end
   
   if (pushCount == dataBitsPerPacket-1) && push
       frameCount(:) = frameCount + 1;
   end
   if (popCount == dataBitsPerPacket-1) && pop
       frameCount(:) = frameCount - 1;
   end

   if push
       if pushCount == dataBitsPerPacket - 1
           pushCount(:) = 0;
       else
           pushCount(:) = pushCount + 1;
       end
   end

   if pop 
       if popCount == dataBitsPerPacket - 1
           popCount(:) = 0;
       else
           popCount(:) = popCount + 1;
       end
   end

   out = frameCount;

end

== matlab function commhdlQPSKTxRxLoopback/Receiver/QPSK Rx/Frequency and Time Synchronizer/Packet Controller/sample discard controller ==
  data: dataIn input; validIn input; dataOut output; startIn input; endIn input; startOut output; endOut output; validOut output
function [dataOut,startOut,endOut,validOut] = controller(dataIn,validIn,startIn,endIn)
%#codegen

   persistent active dataOutReg validOutReg startOutReg endOutReg;
   if isempty(active)
      active  = false;
      dataOutReg = cast(0,'like',dataIn);
      validOutReg = false;
      startOutReg = false;
      endOutReg = false;
   end
   
   dataOut = dataOutReg;
   validOut = validOutReg;
   startOut = startOutReg;
   endOut = endOutReg;
   
   startOutReg = startIn;
   endOutReg = endIn;
   
   if startIn
       active = true;
   end
   
   if active
       dataOutReg(:) = dataIn;
       validOutReg = validIn;
   else
       dataOutReg(:) = 0;
       validOutReg = false;
   end
   
   if endIn
       if active 
           endOutReg = true;
       else
           endOutReg = false;
       end
       active = false;
   end
end

== matlab function commhdlQPSKTxRxLoopback/Receiver/QPSK Rx/Frequency and Time Synchronizer/Symbol Synchronizer/Interpolation Control ==
  data: mu output; Delta input; Underflow output
function [mu,Underflow] = Interpolation_ctrl(Delta)
% Implementation of modulo-1 counter for interpolation control listed in
% Figure 8.4.19 of "Digital Communications - A Discrete-Time Approach"
% by Michael Rice. See design details in Chapter 8.4.3 of the same book.
% 
% Input:
%   Delta - Loop filter output. If loop is in lock, delta would be small
% Output:
%   Underflow - Indicator of counter underflow. This is the strobe signal
%               for downstream processing
%   mu - Difference between actual sampling instant and the optimal instant,
%        between zero and one
%#codegen

% countReg - Counter value delayed by 1 sample
% muReg - The estimated timing error normalized by half QPSK symbols

   mask = fi(1-2^(-10),1,11,10);
   
   persistent countReg underflowReg muReg;
   if isempty(countReg)
       countReg  = fi(0,1,11,10);
       muReg = fi(0,1,11,10);
       underflowReg = false;
   end
   
   
   Underflow = underflowReg;
   mu = muReg;   
   
   
   counter = bitand(mask,countReg)-Delta-fi(0.25,1,11,10); % decrementing counter
   
   % if countReg is a nonnegative number,
   % then mod(countReg,1) equals the fractional part of countReg
   if counter < 0
       underflowReg = true;
       muReg = bitshift(bitand(mask,countReg),2);
       countReg = fi(counter+1,1,11,10);% create underflow to counter
   else
       underflowReg = false;
       countReg = fi(counter,1,11,10);
   end
   


end

== matlab function commhdlQPSKTxRxLoopback/Receiver/QPSK Rx/Frequency and Time Synchronizer/Preamble Detector/Correlator/ThresholdLimiter ==
  settings: fimath=hdlfimath
  data: x input; y output
function y = applyLowerLimit(x)
    % Apply a lower limit to the threshold.
    %#codegen
    
    % Threshold is computed by summing across 63 samples.
    % Set lower limit to be equivalent of all 63 samples
    % having their LSB set to 1 and all others set to 0. 
    lowerLimit = cast(0.01, 'like', x);
    
    if x < lowerLimit
        y = lowerLimit;
    else
        y = x;
    end
end

== matlab function commhdlQPSKTxRxLoopback/Transmitter/Input Data/Message Generator/MATLAB Function ==
  data: enable input; reset input; out output; start output; stop output; valid output; count_out output; msg_count_out output
function [out, start, stop, valid, count_out, msg_count_out] = msggen(enable, reset)

persistent indexCount;
persistent toggle;
persistent msgCount;
persistent msgCountAll;
persistent msgCountBitIndex;

if isempty(indexCount) || isempty(toggle) || isempty(msgCount) || isempty(msgCountBitIndex) || isempty(msgCountAll)
    indexCount = uint32(0);
    msgCount = uint32(1);
    msgCountAll = uint32(1);
    msgCountBitIndex = uint8(0);
    toggle = false;
end

%% Constants
strAscii = dec2bin('ADI Hello World', 8);
msgarray = reshape(strAscii', [1, numel(strAscii)]);
msgbits = logical(msgarray - 48);
msgbitsLen = length(msgbits);

fullMessageLen = uint32(2240-1); % Need the -1 to eat the feedback delay

% Bit counter
% N = 8;% 8-bit counter
% mask = uint32(2^N - 1);
% for k = 1:300
%     msgCount = bitand(msgCount + uint32(1), mask);   % wraps 255 -> 0
% end

%% Logic
if enable && ~reset
    % Set out data
    if indexCount < msgbitsLen % Insert msg
        out = msgbits(indexCount + 1);
        msgCountBitIndex = uint8(0);
    elseif msgCountBitIndex < (8) % Number insert
        out = bitget(msgCount+48, 8-msgCountBitIndex) > 0;
        msgCountBitIndex = msgCountBitIndex + 1;
    else % Toggle bits after message
        out = toggle;
        msgCountBitIndex = uint8(0);
        if toggle
            toggle = false;
        else
            toggle = true;
        end
    end

    % Flags
    start = indexCount == uint32(0);
    stop = indexCount == fullMessageLen;
    valid = true;

    % Counters
    if fullMessageLen == indexCount
        if msgCount >= 9
            msgCount = uint32(1);
        else
            msgCount = msgCount +  1;
            msgCountAll = msgCountAll + 1;
        end
    end
    if indexCount <= fullMessageLen
        indexCount = indexCount + 1;
    end

else % Enable == false

    if reset
        indexCount = uint32(0);
        % msgCount = uint32(0);
        msgCountBitIndex = uint8(0);
        toggle = false;
    end
    out = false;
    start = false;
    stop = false;
    valid = false;
end

if isempty(indexCount)
    count_out = uint32(0);
else
    count_out = indexCount;
end

msg_count_out = msgCountAll;

== matlab function commhdlQPSKTxRxLoopback/Receiver/QPSK Rx/Frequency and Time Synchronizer/Symbol Synchronizer/Rate Handle/FIFO/Validate Input Push Pop/No HDL/MATLAB Function ==
  data: pushFullDiag input; popEmptyDiag input; pushFull input; popEmpty input
function pushPopDiagnostics(pushFullDiag, popEmptyDiag, pushFull, popEmpty)
%#codegen


if(pushFull)
    switch pushFullDiag
        case 2
            warning('Push signal applied on full FIFO');
        case 3
            error('Push signal applied on full FIFO');
        otherwise
    end
end

if(popEmpty)
    switch popEmptyDiag
        case 2
            warning('Pop signal applied on empty FIFO');
        case 3
            error('Pop signal applied on empty FIFO');
        otherwise
    end
end

end
